simulink model "model"  (Simulink 7.3)
settings: Solver=ode3  StartTime=0.0  StopTime=T  FixedStep=dt  RelTol=1e-3
values from neighbouring files (symbols this model uses):
  A = 0.06    [PSO.m]    (also in main.m)
  b = x(2)    [PSO.m]    (also in main.m = 2000)
  f = 2*pi*10    (= 62.8318530718)    [PSO.m]    (also in main.m = 157.079632679)
  g = 9.81    [PSO.m]    (also in main.m)
  k1 = x(1)    [PSO.m]    (also in main.m = 20000)
  k2 = 2e5    (= 200000)    [PSO.m]    (also in main.m)
  m1 = 400    [PSO.m]    (also in main.m)
  m2 = 50    [PSO.m]    (also in main.m)
  x1_0 = - m1*g/k1+x2_0    [PSO.m]    (also in main.m = -0.2182725)
  x2_0 = -(m1+m2)*g/k2    (= -0.0220725)    [PSO.m]    (also in main.m)
settings Model: Creator=adwoznia  LastModifiedBy=adwoznia

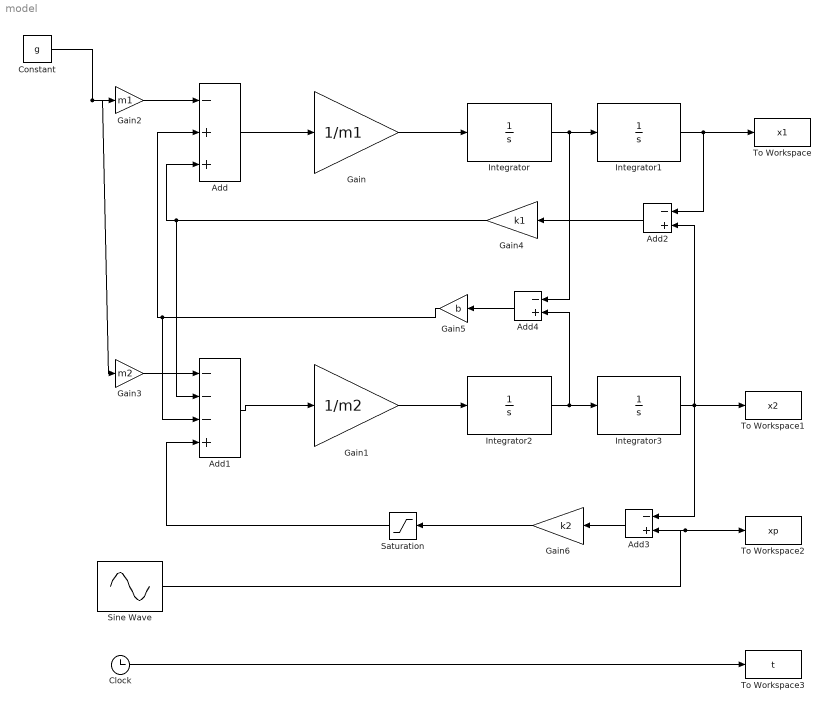
== system model ==
  Add : Sum  Inputs=-++  OutDataType=fixdt(1, 16)  OutScaling=2^-10
  Add1 : Sum  Inputs=---+  OutDataType=fixdt(1, 16)  OutScaling=2^-10
  Add2 : Sum  Inputs=-+  OutDataType=fixdt(1, 16)  OutScaling=2^-10
  Add3 : Sum  Inputs=-+  OutDataType=fixdt(1, 16)  OutScaling=2^-10
  Add4 : Sum  Inputs=-+  OutDataType=fixdt(1, 16)  OutScaling=2^-10
  Clock : Clock
      settings: Decimation=10
  Constant : Constant  Value=g  OutDataType=fixdt(1, 16)  OutScaling=2^0
  Gain : Gain  Gain=1/m1  ParameterDataType=fixdt(1, 16)  ParameterScaling=2^0  OutDataType=fixdt(1, 16)  OutScaling=2^0
  Gain1 : Gain  Gain=1/m2  ParameterDataType=fixdt(1, 16)  ParameterScaling=2^0  OutDataType=fixdt(1, 16)  OutScaling=2^0
  Gain2 : Gain  Gain=m1  ParameterDataType=fixdt(1, 16)  ParameterScaling=2^0  OutDataType=fixdt(1, 16)  OutScaling=2^0
  Gain3 : Gain  Gain=m2  ParameterDataType=fixdt(1, 16)  ParameterScaling=2^0  OutDataType=fixdt(1, 16)  OutScaling=2^0
  Gain4 : Gain  Gain=k1  ParameterDataType=fixdt(1, 16)  ParameterScaling=2^0  OutDataType=fixdt(1, 16)  OutScaling=2^0
  Gain5 : Gain  Gain=b  ParameterDataType=fixdt(1, 16)  ParameterScaling=2^0  OutDataType=fixdt(1, 16)  OutScaling=2^0
  Gain6 : Gain  Gain=k2  ParameterDataType=fixdt(1, 16)  ParameterScaling=2^0  OutDataType=fixdt(1, 16)  OutScaling=2^0
  Integrator : Integrator
  Integrator1 : Integrator  InitialCondition=x1_0
  Integrator2 : Integrator
  Integrator3 : Integrator  InitialCondition=x2_0
  Saturation : Saturate  UpperLimit=Inf  LowerLimit=0  OutDataType=fixdt(1, 16)  OutScaling=2^0
  Sine Wave : Sin  Amplitude=A  Bias=0  Frequency=f  Phase=0  Samples=10  SampleTime=0  Offset=0
  To Workspace : ToWorkspace  VariableName=x1  SampleTime=-1  SaveFormat=Array
  To Workspace1 : ToWorkspace  VariableName=x2  SampleTime=-1  SaveFormat=Array
  To Workspace2 : ToWorkspace  VariableName=xp  SampleTime=-1  SaveFormat=Array
  To Workspace3 : ToWorkspace  VariableName=t  SampleTime=-1  SaveFormat=Array
  wires:
  Add/1 -> Gain/1
  Gain/1 -> Integrator/1
  Integrator/1 -> Integrator1/1, Add4/1
  Add1/1 -> Gain1/1
  Gain1/1 -> Integrator2/1
  Integrator2/1 -> Integrator3/1, Add4/2
  Constant/1 -> Gain3/1, Gain2/1
  Gain3/1 -> Add1/1
  Gain2/1 -> Add/1
  Integrator1/1 -> Add2/1, To Workspace/1
  Integrator3/1 -> Add2/2, Add3/1, To Workspace1/1
  Add2/1 -> Gain4/1
  Gain4/1 -> Add/3, Add1/2
  Gain5/1 -> Add/2, Add1/3
  Add4/1 -> Gain5/1
  Sine Wave/1 -> To Workspace2/1, Add3/2
  Add3/1 -> Gain6/1
  Gain6/1 -> Saturation/1
  Clock/1 -> To Workspace3/1
  Saturation/1 -> Add1/4
